simulink model "SmallSignalLoopSimulation"  (R2025a)
settings: Solver=VariableStepAuto  StartTime=0.0  StopTime=1
undefined symbols (not defined in the file or in its folder): id, vds, vgs
libraries: cstblocks x8
settings Model: Creator=josephderay  LastModifiedBy=josephderay
settings HardwareCC: ProdBitPerLong=64.0  ProdHWDeviceType=Apple->ARM64

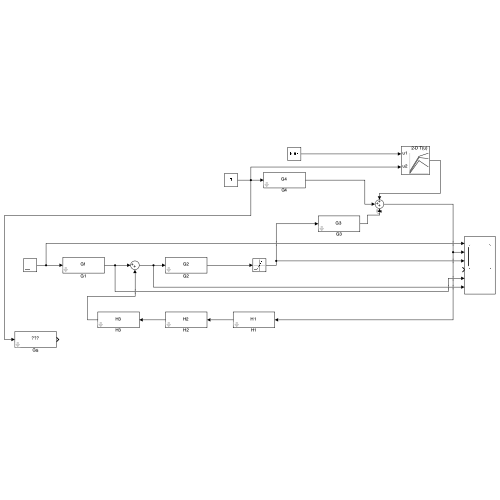
[thumbnail: Simulink's stored preview of the top-level diagram]
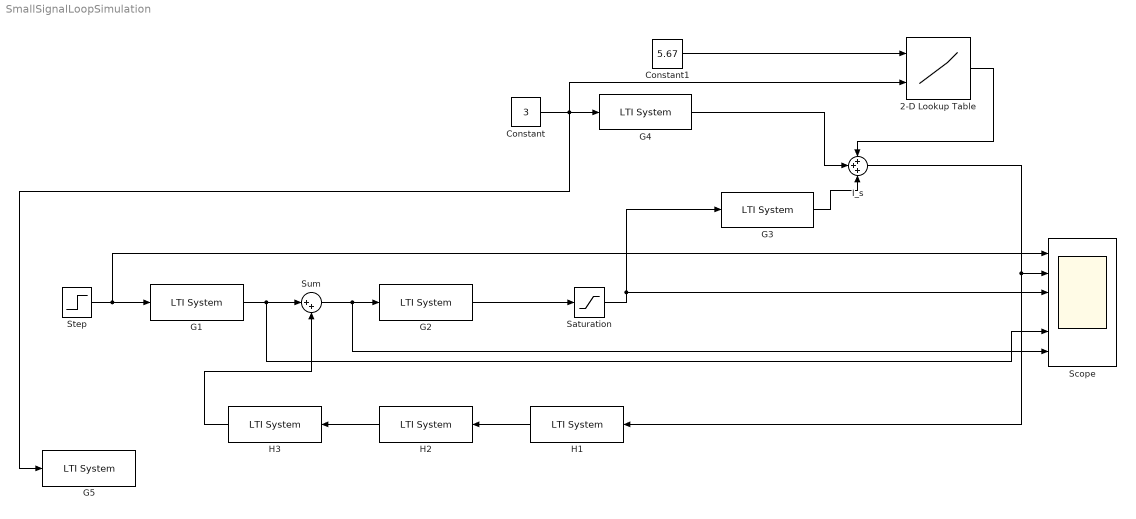
== system SmallSignalLoopSimulation ==
  2-D Lookup Table : Lookup_n-D  BreakpointsForDimension1=vgs  BreakpointsForDimension2=vds  Table=id  InternalRulePriority=Speed  RndMeth=Simplest
      settings: InputPortMap=u0,u1
  Constant : Constant  Value=3
  Constant1 : Constant  Value=5.67
  G1 : cstblocks/LTI System  sys=G1  IC=[]  PadeOrder=0
  G2 : cstblocks/LTI System  sys=G2  IC=[]  PadeOrder=0
  G3 : cstblocks/LTI System  sys=G3  IC=[]  PadeOrder=0
  G4 : cstblocks/LTI System  sys=G4  IC=[]  PadeOrder=0
  G5 : cstblocks/LTI System  sys=G5  IC=[]  PadeOrder=0
  H1 : cstblocks/LTI System  sys=H1  IC=[]  PadeOrder=0
  H2 : cstblocks/LTI System  sys=H2  IC=[]  PadeOrder=0
  H3 : cstblocks/LTI System  sys=H3  IC=[]  PadeOrder=0
  I_s : Sum  Inputs=+++
  Saturation : Saturate  UpperLimit=21.98  LowerLimit=-4.98
  Scope : Scope  NumInputPorts=6
      settings: ActiveDisplayYMinimum=0.58943491115833657  ActiveDisplayYMaximum=3.0409093756582886
  Step : Step  Time=0.4  After=0.705  SampleTime=0
  Sum : Sum  Inputs=|++
  wires:
  G1/1 -> Scope/5, Sum/1
  Step/1 -> Scope/1, G1/1
  H3/1 -> Sum/2
  Sum/1 -> Scope/6, G2/1
  H1/1 -> H2/1
  H2/1 -> H3/1
  I_s/1 -> H1/1, Scope/2
  Constant/1 -> G5/1, G4/1, 2-D Lookup Table/2
  G2/1 -> Saturation/1
  Saturation/1 -> G3/1, Scope/3
  G4/1 -> I_s/2
  G3/1 -> I_s/3
  2-D Lookup Table/1 -> I_s/1
  Constant1/1 -> 2-D Lookup Table/1
